simulink model "RL_sus_quarter_sim"  (R2025a)
settings: Solver=FixedStepAuto  StartTime=0.0  StopTime=20  FixedStep=0.001  RelTol=1e-3
model workspace (MAT data in the model file):
  G0 = Simulink.Parameter
  G0.Value = 0.000256
  G0.Complexity = 'real'
  G0.Dimensions = [1 1]
  G0.DataType = 'auto'
  Q_F = Simulink.Parameter
  Q_F.Value = 0.1
  Q_F.Complexity = 'real'
  Q_F.Dimensions = [1 1]
  Q_F.DataType = 'auto'
  Q_dot_s = Simulink.Parameter
  Q_dot_s.Value = 0.7
  Q_dot_s.Complexity = 'real'
  Q_dot_s.Dimensions = [1 1]
  Q_dot_s.DataType = 'auto'
  Q_dot_s_h = Simulink.Parameter
  Q_dot_s_h.Value = 0.25
  Q_dot_s_h.Complexity = 'real'
  Q_dot_s_h.Dimensions = [1 1]
  Q_dot_s_h.DataType = 'auto'
  Q_dot_u = Simulink.Parameter
  Q_dot_u.Value = 0.001
  Q_dot_u.Complexity = 'real'
  Q_dot_u.Dimensions = [1 1]
  Q_dot_u.DataType = 'auto'
  Q_flec = Simulink.Parameter
  Q_flec.Value = 0.1
  Q_flec.Complexity = 'real'
  Q_flec.Dimensions = [1 1]
  Q_flec.DataType = 'auto'
  Q_flec_t = Simulink.Parameter
  Q_flec_t.Value = 0.1
  Q_flec_t.Complexity = 'real'
  Q_flec_t.Dimensions = [1 1]
  Q_flec_t.DataType = 'auto'
  b_deflec = Simulink.Parameter
  b_deflec.Value = 0.05
  b_deflec.Complexity = 'real'
  b_deflec.Dimensions = [1 1]
  b_deflec.DataType = 'auto'
  b_deflec.DocUnits = 'm'
  bump_height = Simulink.Parameter
  bump_height.Value = 0.02
  bump_height.Complexity = 'real'
  bump_height.Dimensions = [1 1]
  bump_height.DataType = 'auto'
  bump_lenth = Simulink.Parameter
  bump_lenth.Value = 0.5
  bump_lenth.Complexity = 'real'
  bump_lenth.Dimensions = [1 1]
  bump_lenth.DataType = 'auto'
  bump_start = Simulink.Parameter
  bump_start.Value = 1
  bump_start.Complexity = 'real'
  bump_start.Dimensions = [1 1]
  bump_start.DataType = 'auto'
  f0 = Simulink.Parameter
  f0.Value = 0.1
  f0.Complexity = 'real'
  f0.Dimensions = [1 1]
  f0.DataType = 'auto'
  kt = Simulink.Parameter
  kt.Value = 200000
  kt.Complexity = 'real'
  kt.Dimensions = [1 1]
  kt.DataType = 'auto'
  ms = Simulink.Parameter
  ms.Value = 400
  ms.Complexity = 'real'
  ms.Dimensions = [1 1]
  ms.DataType = 'auto'
  n0 = Simulink.Parameter
  n0.Value = 0.1
  n0.Complexity = 'real'
  n0.Dimensions = [1 1]
  n0.DataType = 'auto'
  n1 = Simulink.Parameter
  n1.Value = 0.01
  n1.Complexity = 'real'
  n1.Dimensions = [1 1]
  n1.DataType = 'auto'
  omega_1 = Simulink.Parameter
  omega_1.Value = 2
  omega_1.Complexity = 'real'
  omega_1.Dimensions = [1 1]
  omega_1.DataType = 'auto'
  omega_2 = Simulink.Parameter
  omega_2.Value = 0.15
  omega_2.Complexity = 'real'
  omega_2.Dimensions = [1 1]
  omega_2.DataType = 'auto'
  omega_3 = Simulink.Parameter
  omega_3.Value = 0.15
  omega_3.Complexity = 'real'
  omega_3.Dimensions = [1 1]
  omega_3.DataType = 'auto'
  omega_4 = Simulink.Parameter
  omega_4.Value = 3
  omega_4.Complexity = 'real'
  omega_4.Dimensions = [1 1]
  omega_4.DataType = 'auto'
  ramp_height = Simulink.Parameter
  ramp_height.Value = 0.02
  ramp_height.Complexity = 'real'
  ramp_height.Dimensions = [1 1]
  ramp_height.DataType = 'auto'
  ramp_lenth = Simulink.Parameter
  ramp_lenth.Value = 2
  ramp_lenth.Complexity = 'real'
  ramp_lenth.Dimensions = [1 1]
  ramp_lenth.DataType = 'auto'
  ramp_start = Simulink.Parameter
  ramp_start.Value = 1
  ramp_start.Complexity = 'real'
  ramp_start.Dimensions = [1 1]
  ramp_start.DataType = 'auto'
  sine_amp = Simulink.Parameter
  sine_amp.Value = 0.002
  sine_amp.Complexity = 'real'
  sine_amp.Dimensions = [1 1]
  sine_amp.DataType = 'auto'
  sine_amp.DocUnits = 'm'
  sine_freq = Simulink.Parameter
  sine_freq.Value = 13
  sine_freq.Complexity = 'real'
  sine_freq.Dimensions = [1 1]
  sine_freq.DataType = 'auto'
  sine_freq.DocUnits = 'Hz'
  u = Simulink.Parameter
  u.Value = 25
  u.Complexity = 'real'
  u.Dimensions = [1 1]
  u.DataType = 'auto'
undefined symbols (not defined in the file): Ground, Hook, SH_ADD_new_as_as_xdef
libraries: fl_lib x250, nesl_utility x48, sharedTrackingLibrary x34, dspstat3 x18, simulink x3, deeplib x2, slpidlib x1
(part 1 of 12)
settings Model: PauseTimes=22.92  ParameterArgumentNames=G0,Q_F,Q_dot_s,Q_dot_s_h,Q_dot_u,Q_flec,Q_flec_t,b_deflec,bump_height,bump_lenth,bump_start,omega_1,omega_2,omega_3,omega_4,sine_amp,sine_freq,u  Creator=Asus  LastModifiedBy=Asus
settings RTWCC: GPUComputeCapability=3.5

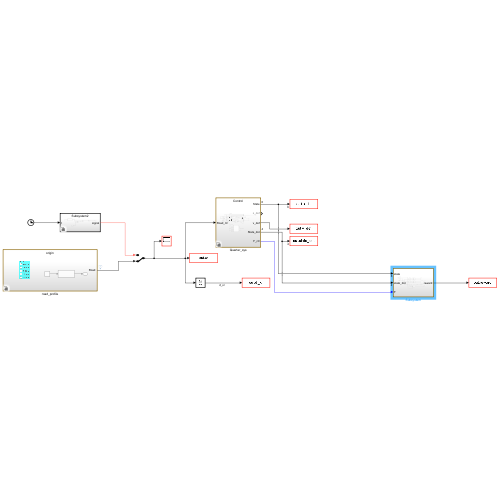
[thumbnail: Simulink's stored preview of the top-level diagram]
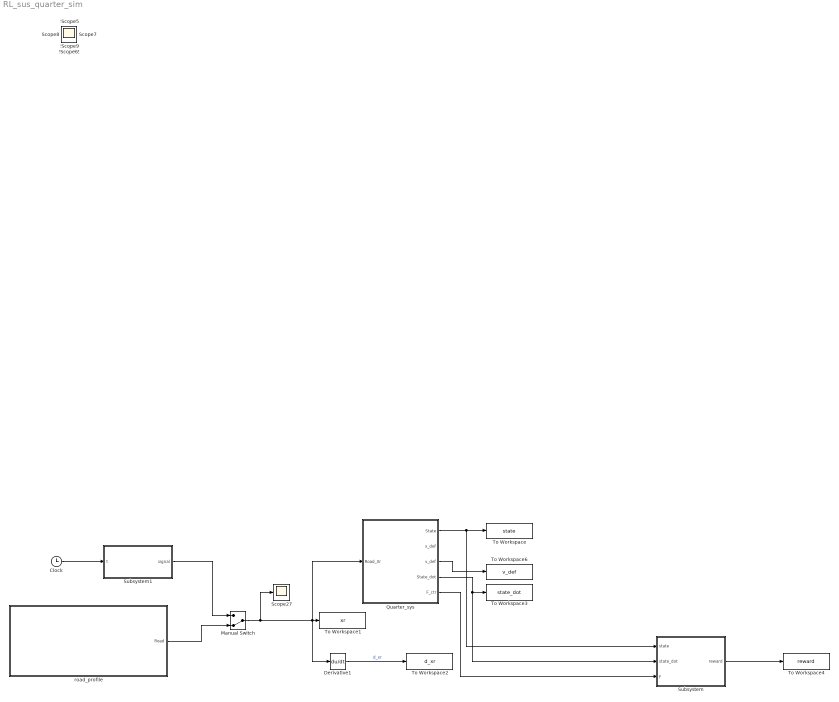
== system RL_sus_quarter_sim ==
  Clock : Clock
  Derivative1 : Derivative
  Manual Switch : ManualSwitch  CurrentSetting=0
  Quarter_sys : Subsystem  Variant=on  VariantControlMode=label  VariantControl=Subsystem  LabelModeActiveChoice=Ctr
  Scope{,1..9,12,27} (12 alike) : Scope
      Scope27 settings: ActiveDisplayYMinimum=-0.005  ActiveDisplayYMaximum=0.045  DataLoggingVariableName=ScopeData4
      Scope settings: ActiveDisplayYMinimum=-0.125  ActiveDisplayYMaximum=1.125
      Scope1 settings: ActiveDisplayYMinimum=-21.6348  ActiveDisplayYMaximum=27.8889
      Scope12 settings: ActiveDisplayYMinimum=-1.43429  ActiveDisplayYMaximum=11.73941  DataLoggingVariableName=ScopeData16
      Scope2 settings: ActiveDisplayYMinimum=-1.25  ActiveDisplayYMaximum=1.25  DataLoggingVariableName=ScopeData2
      Scope3 settings: ActiveDisplayYMinimum=-6.01462  ActiveDisplayYMaximum=2.04507  DataLoggingVariableName=ScopeData3
      Scope5 settings: ActiveDisplayYMinimum=-3.30691  ActiveDisplayYMaximum=4.00872  DataLoggingVariableName=ScopeData2
      Scope6 settings: ActiveDisplayYMinimum=-0.24558  ActiveDisplayYMaximum=1.31955
      Scope7 settings: ActiveDisplayYMinimum=-0.13437  ActiveDisplayYMaximum=0.12404
      Scope8 settings: ActiveDisplayYMinimum=-3.52473  ActiveDisplayYMaximum=3.04502  DataLoggingVariableName=ScopeData2
      Scope9 settings: ActiveDisplayYMinimum=-2441.21956  ActiveDisplayYMaximum=2573.78427  DataLoggingVariableName=ScopeData2
  Subsystem : Subsystem
  Subsystem1 : Subsystem  Variant=on  VariantControlMode=label  VariantControl=Subsystem1  LabelModeActiveChoice=variant freq amp
  To Workspace : ToWorkspace  VariableName=state  SampleTime=-1
      settings: Save2DSignal=2-D array (concatenate along first dimension)
  To Workspace1 : ToWorkspace  VariableName=xr  SampleTime=-1
      settings: Save2DSignal=2-D array (concatenate along first dimension)
  To Workspace2 : ToWorkspace  VariableName=d_xr  SampleTime=-1
      settings: Save2DSignal=2-D array (concatenate along first dimension)
  To Workspace3 : ToWorkspace  VariableName=state_dot  SampleTime=-1
      settings: Save2DSignal=2-D array (concatenate along first dimension)
  To Workspace4 : ToWorkspace  VariableName=reward  SampleTime=-1
      settings: Save2DSignal=2-D array (concatenate along first dimension)
  To Workspace6 : ToWorkspace  VariableName=v_def  SampleTime=-1
      settings: Save2DSignal=2-D array (concatenate along first dimension)
  road_profile : Subsystem  Variant=on  VariantControlMode=label  LabelModeActiveChoice=OriginRoad
  wires:
  Manual Switch/1 -> Quarter_sys/1(Road_Xr), To Workspace1/1, Derivative1/1, Scope27/1
  Derivative1/1 -> To Workspace2/1  "d_xr"
  Quarter_sys/3(v_def) -> To Workspace6/1
  Quarter_sys/4(State_dot) -> Subsystem/2(state_dot), To Workspace3/1
  Quarter_sys/1(State) -> Subsystem/1(state), To Workspace/1
  Clock/1 -> Subsystem1/1(t)
  Subsystem1/1(signal) -> Manual Switch/1
  road_profile/1("Road ") -> Manual Switch/2
  Subsystem/1(reward) -> To Workspace4/1
  Quarter_sys/5(F_ctr) -> Subsystem/3(F)

== system RL_sus_quarter_sim/Quarter_sys ==
  Road_Xr : Inport
  Control : Subsystem  VariantControl=Ctr
  Passive : Subsystem  VariantControl=Passive
  State : Outport
  x_def : Outport  Port=2
  v_def : Outport  Port=3
  State_dot : Outport  Port=4
  F_ctr : Outport  Port=5

== system RL_sus_quarter_sim/Subsystem ==
  state : Inport
  state_dot : Inport  Port=2
  F : Inport  Port=3
  Abs : Abs  SaturateOnIntegerOverflow=off
  Abs1 : Abs  SaturateOnIntegerOverflow=off
  Add2 : Sum  Inputs=+++
  Add4 : Sum  Inputs=----
  Constant2 : Constant  Value=0
  Constant3 : Constant  Value=-500
  Floor : Rounding
  Gain : Gain  Gain=Q_dot_s
  Gain10 : Gain  Gain=-1
  Gain11 : Gain  Gain=Q_dot_s_h
  Gain3 : Gain  Gain=1/omega_1
  Gain4 : Gain  Gain=1/omega_2
  Gain5 : Gain  Gain=Q_flec
  Gain6 : Gain  Gain=1/omega_3
  Gain7 : Gain  Gain=Q_flec_t
  Gain8 : Gain  Gain=1/omega_4
  Gain9 : Gain  Gain=Q_F
  Memory : Memory
  N2kN : Gain  Gain=1/1000
  Selector : Selector  InputPortWidth=4  IndexOptions=Index vector (dialog)  Indices=[2]  OutputSizes=1
  Selector1 : Selector  InputPortWidth=6  IndexOptions=Index vector (dialog)  Indices=[6]  OutputSizes=1
  Selector2 : Selector  InputPortWidth=6  IndexOptions=Index vector (dialog)  Indices=[5]  OutputSizes=1
  Square{,1..3} (4 alike) : Math  Operator=square
  Switch : Switch  Criteria=u2 > Threshold  Threshold=b_deflec  SaturateOnIntegerOverflow=off  InputSameDT=off
  reward : Outport
  wires:
  Gain5/1 -> Add4/1  "reward_flec"
  Gain6/1 -> Square2/1
  Constant3/1 -> Switch/1
  Abs1/1 -> Switch/2
  Floor/1 -> Gain11/1
  Gain8/1 -> Square3/1
  Abs/1 -> Floor/1
  F/1 -> Memory/1
  Gain4/1 -> Square1/1
  Square3/1 -> Gain9/1
  Square/1 -> Gain/1
  Gain3/1 -> Square/1
  state_dot/1 -> Selector/1
  Selector/1 -> Gain3/1, Abs/1  "as"
  state/1 -> Selector1/1, Selector2/1
  Gain/1 -> Add4/2  "reward_accs"
  Memory/1 -> N2kN/1
  Gain10/1 -> Add2/2  "hard_reward"
  Switch/1 -> Add2/3
  Constant2/1 -> Switch/3
  Square2/1 -> Gain7/1
  Add4/1 -> Add2/1  "soft_reward"
  Gain11/1 -> Gain10/1
  Gain9/1 -> Add4/4  "reward_F"
  Gain7/1 -> Add4/3  "reward_tire"
  Selector2/1 -> Gain6/1  "x_tire"
  Selector1/1 -> Gain4/1, Abs1/1  "x_def"
  Add2/1 -> reward/1  "reward"
  N2kN/1 -> Gain8/1
  Square1/1 -> Gain5/1

== system RL_sus_quarter_sim/Subsystem1 ==
  t : Inport
  Subsystem1 : Subsystem  VariantControl=variant freq
  Subsystem2 : Subsystem  VariantControl=variant freq amp
  signal : Outport

== system RL_sus_quarter_sim/road_profile ==
  note: 1) Add Subsystem or Model blocks as valid variant choices.
      | 2) You cannot connect blocks at this level. At simulation, connectivity is automatically
      | determined, based on the active variant and port name matching.
  Subsystem : Subsystem  VariantControl=Look table
  gp : Subsystem  VariantControl=GpSample
  origin : Subsystem  VariantControl=OriginRoad
  "Road " : Outport

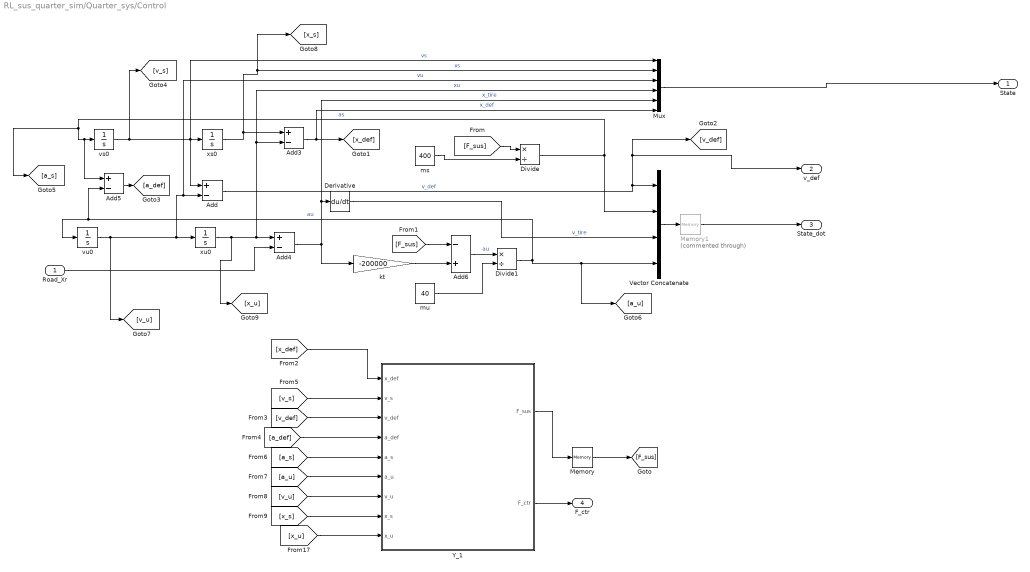
== system RL_sus_quarter_sim/Quarter_sys/Control ==
  Road_Xr : Inport
  Add{,3..5} (4 alike) : Sum  Inputs=+-
  Add6 : Sum  Inputs=-+
  Derivative : Derivative
  Divide : Product  Inputs=*/
  Divide1 : Product  Inputs=*/
  Memory : Memory
  Memory1 : Memory  Commented=through
  Mux : Mux  Inputs=6
  Vector Concatenate : Concatenate  NumInputs=4
  Y_1 : Subsystem  Variant=on  VariantControlMode=label  VariantControl=Subsystem  LabelModeActiveChoice=RL_model_imp_force
  kt : Gain  Gain=-200000
  ms : Constant  Value=400
  mu : Constant  Value=40
  vs0 : Integrator
  vu0 : Integrator
  xs0 : Integrator
  xu0 : Integrator
  State : Outport
  v_def : Outport  Port=2
  State_dot : Outport  Port=3
  F_ctr : Outport  Port=4
  wires:
  Y_1/1(F_sus) -> Memory/1
  [a_def] -> Y_1/4(a_def)
  [v_def] -> Y_1/3(v_def)
  [x_def] -> Y_1/1(x_def)
  Add5/1 -> [a_def]
  [F_sus] -> Add6/1
  Add4/1 -> Derivative/1, Mux/5, kt/1  "x_tire"
  kt/1 -> Add6/2
  vu0/1 -> Add/2, Mux/3, xu0/1, [v_u]  "vu"
  xu0/1 -> [x_u], Add3/2, Mux/4, Add4/1  "xu"
  Divide1/1 -> [a_u], Vector Concatenate/4, vu0/1, Add5/2  "au"
  Add/1 -> v_def/1, [v_def], Vector Concatenate/1  "v_def"
  [F_sus] -> Divide/1
  Vector Concatenate/1 -> Memory1/1
  ms/1 -> Divide/2
  vs0/1 -> [v_s], Add/1, Mux/1, xs0/1  "vs"
  Divide/1 -> [a_s], vs0/1, Add5/1, Vector Concatenate/2  "as"
  xs0/1 -> Add3/1, [x_s], Mux/2  "xs"
  Derivative/1 -> Vector Concatenate/3  "v_tire"
  Add3/1 -> Mux/6, [x_def]  "x_def"
  Add6/1 -> Divide1/1  "au"
  mu/1 -> Divide1/2
  Mux/1 -> State/1
  Road_Xr/1 -> Add4/2
  Memory1/1 -> State_dot/1
  [v_s] -> Y_1/2(v_s)
  [a_s] -> Y_1/5(a_s)
  Memory/1 -> [F_sus]
  [a_u] -> Y_1/6(a_u)
  [v_u] -> Y_1/7(v_u)
  [x_s] -> Y_1/8(x_s)
  [x_u] -> Y_1/9(x_u)
  Y_1/2(F_ctr) -> F_ctr/1

== system RL_sus_quarter_sim/Quarter_sys/Passive ==
  Road_Xr : Inport
  Add{,3..5} (4 alike) : Sum  Inputs=+-
  Add6 : Sum  Inputs=-+
  Derivative : Derivative
  Divide : Product  Inputs=*/
  Divide1 : Product  Inputs=*/
  Memory1 : Memory  Commented=through
  Mux : Mux
  Vector Concatenate : Concatenate  NumInputs=4
  Y_1 : Subsystem  Variant=on  VariantControlMode=label  VariantControl=Subsystem  LabelModeActiveChoice=SkyHook
  kt : Gain  Gain=-200000
  ms : Constant  Value=400
  mu : Constant  Value=40
  vs0 : Integrator
  vu0 : Integrator
  xs0 : Integrator
  xu0 : Integrator
  State : Outport
  x_def : Outport  Port=2
  v_def : Outport  Port=3
  State_dot : Outport  Port=4
  wires:
  Memory1/1 -> State_dot/1
  Road_Xr/1 -> Add4/2
  Mux/1 -> State/1
  mu/1 -> Divide1/2
  Add6/1 -> Divide1/1  "au"
  Add3/1 -> [x_def], x_def/1  "x_def"
  Derivative/1 -> Vector Concatenate/3  "v_tire"
  xs0/1 -> Mux/2, Add3/1  "xs"
  Divide/1 -> Vector Concatenate/2, Add5/1, vs0/1  "as"
  vs0/1 -> xs0/1, Mux/1, Add/1  "vs"
  ms/1 -> Divide/2
  Vector Concatenate/1 -> Memory1/1
  [F_sus] -> Divide/1
  Add/1 -> Vector Concatenate/1, [v_def], v_def/1  "v_def"
  Divide1/1 -> Add5/2, vu0/1, Vector Concatenate/4  "au"
  xu0/1 -> Add4/1, Mux/4, Add3/2  "xu"
  vu0/1 -> xu0/1, Mux/3, Add/2  "vu"
  kt/1 -> Add6/2
  Add4/1 -> kt/1, Derivative/1  "x_tire"
  [F_sus] -> Add6/1
  Add5/1 -> [a_def]
  [x_def] -> Y_1/1(x_def)
  [v_def] -> Y_1/2(v_def)
  [a_def] -> Y_1/3(a_def)
  Y_1/1(F_sus) -> [F_sus]

== system RL_sus_quarter_sim/Subsystem1/Subsystem1 ==
  t : Inport
  MATLAB Function4 : MATLAB Function  TreatAsAtomicUnit=on
  signal : Outport
  wires:
  MATLAB Function4/1(signal) -> signal/1
  t/1 -> MATLAB Function4/1(t)

== system RL_sus_quarter_sim/Subsystem1/Subsystem2 ==
  t : Inport
  Add : Sum
  Constant : Constant
  Gain : Gain  Gain=0.01
  MATLAB Function3 : MATLAB Function  TreatAsAtomicUnit=on  SystemSampleTime=0.001
  Manual Switch : ManualSwitch
  signal : Outport
  wires:
  t/1 -> MATLAB Function3/1(t)
  MATLAB Function3/1(signal) -> Manual Switch/1, Add/1
  Manual Switch/1 -> Gain/1
  Add/1 -> Manual Switch/2
  Constant/1 -> Add/2
  Gain/1 -> signal/1
